simulink model "PI_antiwindup_filtro"  (R2023a)
settings: Solver=VariableStepAuto  StartTime=0.0  StopTime=500.0  RelTol=1e-3
libraries: cstblocks x1
settings Model: Creator=vitor  LastModifiedBy=vitor

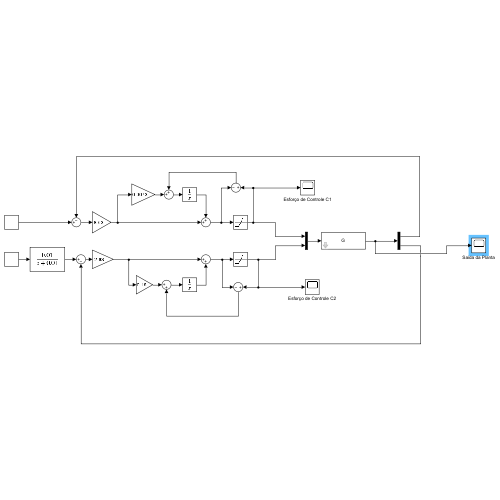
[thumbnail: Simulink's stored preview of the top-level diagram]
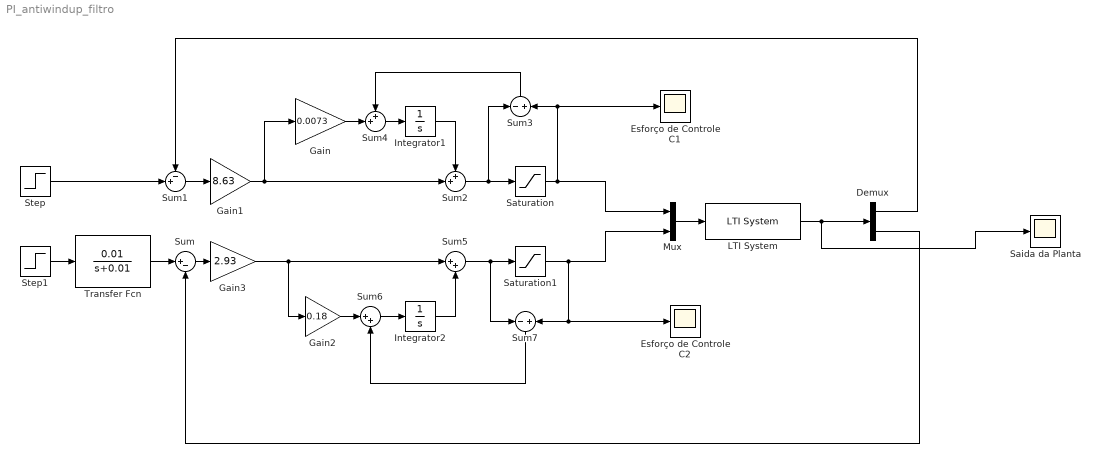
== system PI_antiwindup_filtro ==
  Demux : Demux  Outputs=2
  Esforço de Controle C1 : Scope
  Esforço de Controle C2 : Scope
  Gain : Gain  Gain=0.0073
  Gain1 : Gain  Gain=8.63
  Gain2 : Gain  Gain=0.18
  Gain3 : Gain  Gain=2.93
  Integrator1 : Integrator
  Integrator2 : Integrator
  LTI System : cstblocks/LTI System  sys=G  IC=[]
  Mux : Mux  Inputs=2
  Saida da Planta : Scope
  Saturation : Saturate  UpperLimit=3.33  LowerLimit=0
  Saturation1 : Saturate  UpperLimit=3.35  LowerLimit=0
  Step : Step  Time=10  SampleTime=0
  Step1 : Step  Time=0  SampleTime=0
  Sum : Sum  Inputs=|+-
  Sum1 : Sum  Inputs=-+|
  Sum2 : Sum  Inputs=++|
  Sum3 : Sum  Inputs=-|+
  Sum4 : Sum  Inputs=++|
  Sum5 : Sum  Inputs=|++
  Sum6 : Sum  Inputs=|++
  Sum7 : Sum  Inputs=-|+
  Transfer Fcn : TransferFcn  Numerator=[0.01]  Denominator=[1 0.01]
  wires:
  Demux/1 -> Sum1/1
  Step/1 -> Sum1/2
  LTI System/1 -> Saida da Planta/1, Demux/1
  Mux/1 -> LTI System/1
  Demux/2 -> Sum/2
  Gain1/1 -> Gain/1, Sum2/2
  Sum1/1 -> Gain1/1
  Integrator1/1 -> Sum2/1
  Saturation/1 -> Esforço de Controle C1/1, Sum3/2, Mux/1
  Gain/1 -> Sum4/2
  Sum4/1 -> Integrator1/1
  Sum3/1 -> Sum4/1
  Sum2/1 -> Sum3/1, Saturation/1
  Sum6/1 -> Integrator2/1
  Gain2/1 -> Sum6/1
  Saturation1/1 -> Sum7/2, Esforço de Controle C2/1, Mux/2
  Sum5/1 -> Sum7/1, Saturation1/1
  Integrator2/1 -> Sum5/2
  Gain3/1 -> Sum5/1, Gain2/1
  Sum7/1 -> Sum6/2
  Sum/1 -> Gain3/1
  Step1/1 -> Transfer Fcn/1
  Transfer Fcn/1 -> Sum/1
